simulink model "ask_pe_est"  (Simulink 8.7)
settings: Solver=FixedStepDiscrete  SolverMode=SingleTasking  StartTime=0.0  StopTime=5  FixedStep=1/100000  RelTol=1e-3  AbsTol=1e-6
libraries: commchan3 x1, commsink2 x1, commfilt2 x1, dspsrcs4 x1
settings Model: Creator=amoura  LastModifiedBy=Artur Moura
settings DataIOCC: LimitDataPoints=off  SignalLoggingSaveFormat=ModelDataLogs
settings OptimizationCC: BlockReduction=off  BooleanDataType=off  ExpressionDepthLimit=2147483647  InitFltsAndDblsToZero=on
settings DebuggingCC: SaveWithParameterizedLinksMsg=none  SignalResolutionControl=TryResolveAllWithWarning  MultiTaskDSMMsg=warning  MultiTaskCondExecSysMsg=none  FcnCallInpInsideContextMsg=UseLocalSettings  StateNameClashWarn=warning
settings HardwareCC: TargetUnknown=on
settings RTWCC: TemplateMakefile=grt_unix.tmf
settings GRTTargetCC: TargetFcnLib=ansi_tfl_tmw.mat  ModelReferenceCompliant=off  CombineOutputUpdateFcns=off  MatFileLogging=off  GRTInterface=on

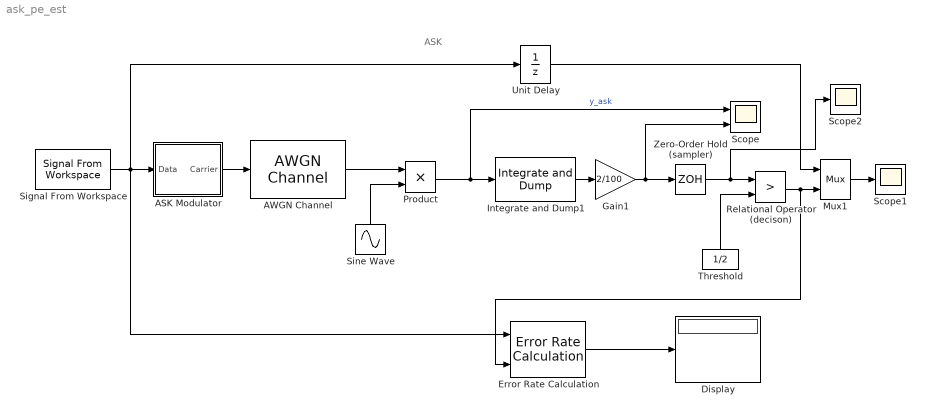
== system ask_pe_est ==
  note: ASK
  ASK Modulator : Subsystem
  AWGN Channel : commchan3/AWGN Channel  InputProcessing=Inherited (this choice will be removed - see release notes)  seed=67  noiseMode=Variance from mask  EbNodB=10  EsNodB=10  SNRdB=10  bitsPerSym=1  Ps=1  Tsym=1  variance=2.5
  Display : Display
  Error Rate Calculation : commsink2/Error Rate Calculation  N=1  st_delay=0  cp_mode=Entire frame  subframe=[]  PMode=Port  WsName=ErrorVec  RsMode2=off  stop=off  numErr=100  maxBits=1e6
  Gain1 : Gain  Gain=2/100  SampleTime=1/100000  SaturateOnIntegerOverflow=on  OutDataTypeStr=Inherit: Same as input  ParamDataTypeStr=Inherit: Same as input
  Integrate and Dump1 : commfilt2/Integrate and Dump  obssamples=100  offsetsamples=1  nodump=on  roundingMode=Floor  overflowMode=off  outputDataTypeStr=Inherit: Same as accumulator  outputLastDataTypeStr=Inherit: Same as accumulator
  Mux1 : Mux  Inputs=2
  Product : Product  SampleTime=1/100000  SaturateOnIntegerOverflow=on  RndMeth=Zero  InputSameDT=on  OutDataTypeStr=Inherit: Same as first input
  Relational Operator (decison) : RelationalOperator  Operator=>  SampleTime=1/1000  InputSameDT=on
  Scope : Scope  NumInputPorts=2
  Scope1 : Scope
  Scope2 : Scope
  Signal From Workspace : dspsrcs4/Signal From Workspace  X=randi([0 1],10000,1)  Ts=1/1000  nsamps=1  OutputAfterFinalValue=Cyclic repetition  ignoreOrWarnInputAndFrameLengths=off  OutputFrames=on
  Sine Wave : Sin  Frequency=2*pi*10000  SampleTime=0
  Threshold : Constant  Value=1/2
  Unit Delay : UnitDelay  SampleTime=1/1000
  Zero-Order Hold (sampler) : ZeroOrderHold  SampleTime=1/1000
  wires:
  Relational Operator (decison)/1 -> Mux1/2, Error Rate Calculation/2
  Sine Wave/1 -> Product/2
  ASK Modulator/1(Carrier) -> AWGN Channel/1
  Zero-Order Hold (sampler)/1 -> Relational Operator (decison)/1, Scope2/1
  Threshold/1 -> Relational Operator (decison)/2
  Product/1 -> Integrate and Dump1/1, Scope/1  "y_ask"
  Mux1/1 -> Scope1/1
  Signal From Workspace/1 -> ASK Modulator/1(Data), Unit Delay/1, Error Rate Calculation/1
  Unit Delay/1 -> Mux1/1
  AWGN Channel/1 -> Product/1
  Error Rate Calculation/1 -> Display/1
  Integrate and Dump1/1 -> Gain1/1
  Gain1/1 -> Zero-Order Hold (sampler)/1, Scope/2

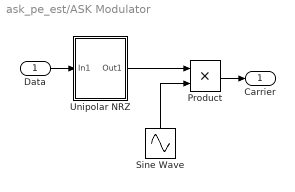
== system ask_pe_est/ASK Modulator ==
  Data : Inport
  Product : Product  SaturateOnIntegerOverflow=on  RndMeth=Zero  InputSameDT=on  OutDataTypeStr=Inherit: Same as first input
  Sine Wave : Sin  Frequency=2*pi*10000  SampleTime=0
  Unipolar NRZ : Subsystem  mask(Unipolar NRZ){}
      mask help:
      | This block encodes a signal into the unipolar NRZ line code
      |
      | The output values are +1 for a nonzero input and zero otherwise.
      mask Display: disp('Unipolar\nNRZ')
  Carrier : Outport  InitialOutput=0
  wires:
  Sine Wave/1 -> Product/2
  Unipolar NRZ/1(Out1) -> Product/1
  Data/1 -> Unipolar NRZ/1(In1)
  Product/1 -> Carrier/1

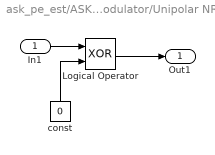
== system ask_pe_est/ASK Modulator/Unipolar NRZ ==
  In1 : Inport
  Logical Operator : Logic  Operator=XOR
  const : Constant  Value=0
  Out1 : Outport  InitialOutput=0
  wires:
  const/1 -> Logical Operator/2
  In1/1 -> Logical Operator/1
  Logical Operator/1 -> Out1/1
